simulink subsystem "darm_mechanics"  (R2021a)
settings: Solver=VariableStepAuto  StartTime=0.0  StopTime=10.0  RelTol=1e-3
undefined symbols (not defined in the file): darm, darm_knm, X, Y, Z
libraries: sm_lib x97, darm_library x77
(part 2 of 5)

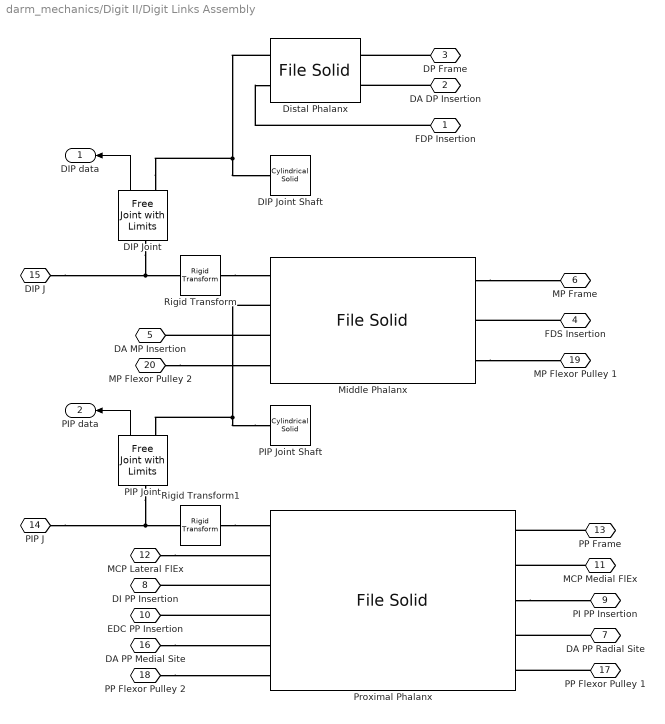
== system darm_mechanics/Digit II/Digit Links Assembly ==
  DIP Joint : darm_library/Free Joint with Limits  joint=digit.dip_joint
  DIP Joint Shaft : sm_lib/Body Elements/Cylindrical Solid  GraphicAmbientColor=[0.15 0.15 0.15 1.0]  BasedOnType=Density  CenterOfMass=[0 0 0]  CenterOfMassUnits=m  GraphicDiffuseColor=[0.5 0.5 0.5]  CylinderLength=digit.dip_joint_shaft_length  CylinderLengthUnits=m  CylinderRadius=digit.dip_joint_shaft_radius  CylinderRadiusUnits=m  Density=darm.link_density  DensityUnits=kg/m^3  DoExposeReferenceFrame=on  GraphicEmissiveColor=[0.0 0.0 0.0 1.0]  ExportEntireGeometry=off  SerializedFrames=<Frames/>  MarkerShape=Sphere  MarkerSize=10  GraphicType=FromGeometry  InertiaType=CalculateFromGeometry  Mass=1  MassUnits=kg  MomentsOfInertia=[1 1 1]  MomentsOfInertiaUnits=kg*m^2  GraphicOpacity=1.0  ProductsOfInertia=[0 0 0]  ProductsOfInertiaUnits=kg*m^2  GraphicShininess=75  GraphicSpecularColor=[0.5 0.5 0.5 1.0]  GraphicVisPropType=SimpleVisualProperties
  Distal Phalanx : sm_lib/Body Elements/File Solid  ExtGeomFileName=C:\Users\Daniel Adejumo\Documents\MATLAB\DARM\Geometry Models and FEA\Models\CAD\Phalanges\Phalanges II\Distal Phalanx II.step  UnitType=FromFile  ExtGeomFileUnits=m  StepReaderType=HEX  ExportConvexHullGeometry=off  InertiaType=CalculateFromGeometry  Mass=1  MassUnits=kg  CenterOfMass=[0 0 0]  CenterOfMassUnits=m  MomentsOfInertia=[1 1 1]  MomentsOfInertiaUnits=kg*m^2  ProductsOfInertia=[0 0 0]  ProductsOfInertiaUnits=kg*m^2  BasedOnType=Density  Density=darm.link_density  DensityUnits=kg/m^3  DoExposeReferenceFrame=on  SerializedFrames=<Frames><Frame><Id>Frame1</Id><Value><Name>J</Name><Origin><Source>ReferenceFrame</Source><FeatureName></FeatureName></Origin><PrimaryAxis><DefinedDirection>+Z</DefinedDirection><Source>ReferenceFrame</Source><SourceDirection>+X</SourceDirection><FeatureName></FeatureName></PrimaryAxis><SecondaryAxis><DefinedDirection>+X</DefinedDirection><Source>ReferenceFrame</Source><SourceDirection>-Z</SourceDirection><FeatureName></FeatureName></SecondaryAxis></Value></Frame><Frame><Id>Frame2</Id><Value><Name>FDP M</Name><Origin><Source>GeometricFeature</Source><FeatureName>circular curve 129</FeatureName></Origin><PrimaryAxis><DefinedDirection>+Z</DefinedDirection><Source>ReferenceFrame</Source><SourceDirection>+Z</SourceDirection><FeatureName></FeatureName></PrimaryAxis><SecondaryAxis><DefinedDirection>+X</DefinedDirection><Source>ReferenceFrame</Source><SourceDirection>+X</SourceDirection><FeatureName></FeatureName></SecondaryAxis></Value></Frame><Frame><Id>Frame3</Id><Value><Name>ED M</Name><Origin><Source>GeometricFeature</Source><FeatureName>circular curve 131</FeatureName></Origin><PrimaryAxis><DefinedDirection>+Z</DefinedDirection><Source>ReferenceFrame</Source><SourceDirection>+Z</SourceDirection><FeatureName></FeatureName></PrimaryAxis><SecondaryAxis><DefinedDirection>+X</DefinedDirection><Source>ReferenceFrame</Source><SourceDirection>+X</SourceDirection><FeatureName></FeatureName></SecondaryAxis></Value></Frame></Frames>  GraphicType=FromGeometry  MarkerShape=Sphere  MarkerSize=10  GraphicVisPropType=SimpleVisualProperties  GraphicDiffuseColor=[0.5 0.5 0.5]  GraphicSpecularColor=[0.5 0.5 0.5 1.0]  GraphicAmbientColor=[0.15 0.15 0.15 1.0]  GraphicEmissiveColor=[0.0 0.0 0.0 1.0]  GraphicShininess=75  GraphicOpacity=1.0
  Middle Phalanx : sm_lib/Body Elements/File Solid  ExtGeomFileName=C:\Users\Daniel Adejumo\Documents\MATLAB\DARM\Geometry Models and FEA\Models\CAD\Phalanges\Phalanges II\Middle Phalanx II.step  UnitType=FromFile  ExtGeomFileUnits=m  StepReaderType=HEX  ExportConvexHullGeometry=off  InertiaType=CalculateFromGeometry  Mass=1  MassUnits=kg  CenterOfMass=[0 0 0]  CenterOfMassUnits=m  MomentsOfInertia=[1 1 1]  MomentsOfInertiaUnits=kg*m^2  ProductsOfInertia=[0 0 0]  ProductsOfInertiaUnits=kg*m^2  BasedOnType=Density  Density=darm.link_density  DensityUnits=kg/m^3  DoExposeReferenceFrame=on  SerializedFrames=<Frames><Frame><Id>Frame2</Id><Value><Name>DIP J*</Name><Origin><Source>GeometricFeature</Source><FeatureName>circular curve 214</FeatureName></Origin><PrimaryAxis><DefinedDirection>+Z</DefinedDirection><Source>ReferenceFrame</Source><SourceDirection>+X</SourceDirection><FeatureName></FeatureName></PrimaryAxis><SecondaryAxis><DefinedDirection>+X</DefinedDirection><Source>ReferenceFrame</Source><SourceDirection>-Z</SourceDirection><FeatureName></FeatureName></SecondaryAxis></Value></Frame><Frame><Id>Frame3</Id><Value><Name>PIP J</Name><Origin><Source>ReferenceFrame</Source><FeatureName></FeatureName></Origin><PrimaryAxis><DefinedDirection>+Z</DefinedDirection><Source>ReferenceFrame</Source><SourceDirection>+X</SourceDirection><FeatureName></FeatureName></PrimaryAxis><SecondaryAxis><DefinedDirection>+X</DefinedDirection><Source>ReferenceFrame</Source><SourceDirection>-Z</SourceDirection><FeatureName></FeatureName></SecondaryAxis></Value></Frame><Frame><Id>Frame4</Id><Value><Name>FDS M</Name><Origin><Source>GeometricFeature</Source><FeatureName>circular curve 209</FeatureName></Origin><PrimaryAxis><DefinedDirection>+Z</DefinedDirection><Source>ReferenceFrame</Source><SourceDirection>+Z</SourceDirection><FeatureName></FeatureName></PrimaryAxis><SecondaryAxis><DefinedDirection>+X</DefinedDirection><Source>ReferenceFrame</Source><SourceDirection>+X</SourceDirection><FeatureName></FeatureName></SecondaryAxis></Value></Frame><Frame><Id>Frame5</Id><Value><Name>ED M</Name><Origin><Source>GeometricFeature</Source><FeatureName>circular curve 205</FeatureName></Origin><PrimaryAxis><DefinedDirection>+Z</DefinedDirection><Source>ReferenceFrame</Source><SourceDirection>+Z</SourceDirection><FeatureName></FeatureName></PrimaryAxis><SecondaryAxis><DefinedDirection>+X</DefinedDirection><Source>ReferenceFrame</Source><SourceDirection>+X</SourceDirection><FeatureName></FeatureName></SecondaryAxis></Value></Frame><Frame><Id>Frame6</Id><Value><Name>Flexor Pulley 1</Name><Origin><Source>GeometricFeature</Source><FeatureName>point 616</FeatureName></Origin><PrimaryAxis><DefinedDirection>+Z</DefinedDirection><Source>ReferenceFrame</Source><SourceDirection>+Z</SourceDirection><FeatureName></FeatureName></PrimaryAxis><SecondaryAxis><DefinedDirection>+X</DefinedDirection><Source>ReferenceFrame</Source><SourceDirection>+X</SourceDirection><FeatureName></FeatureName></SecondaryAxis></Value></Frame><Frame><Id>Frame7</Id><Value><Name>Flexor Pulley 2</Name><Origin><Source>GeometricFeature</Source><FeatureName>segment 75</FeatureName></Origin><PrimaryAxis><DefinedDirection>+Z</DefinedDirection><Source>ReferenceFrame</Source><SourceDirection>+Z</SourceDirection><FeatureName></FeatureName></PrimaryAxis><SecondaryAxis><DefinedDirection>+X</DefinedDirection><Source>ReferenceFrame</Source><SourceDirection>+X</SourceDirection><FeatureName></FeatureName></SecondaryAxis></Value></Frame></Frames>  GraphicType=FromGeometry  MarkerShape=Sphere  MarkerSize=10  GraphicVisPropType=SimpleVisualProperties  GraphicDiffuseColor=[0.5 0.5 0.5]  GraphicSpecularColor=[0.5 0.5 0.5 1.0]  GraphicAmbientColor=[0.15 0.15 0.15 1.0]  GraphicEmissiveColor=[0.0 0.0 0.0 1.0]  GraphicShininess=75  GraphicOpacity=1.0
  PIP Joint : darm_library/Free Joint with Limits  joint=digit.pip_joint
  PIP Joint Shaft : sm_lib/Body Elements/Cylindrical Solid  GraphicAmbientColor=[0.15 0.15 0.15 1.0]  BasedOnType=Density  CenterOfMass=[0 0 0]  CenterOfMassUnits=m  GraphicDiffuseColor=[0.5 0.5 0.5]  CylinderLength=digit.pip_joint_shaft_length  CylinderLengthUnits=m  CylinderRadius=digit.pip_joint_shaft_radius  CylinderRadiusUnits=m  Density=darm.link_density  DensityUnits=kg/m^3  DoExposeReferenceFrame=on  GraphicEmissiveColor=[0.0 0.0 0.0 1.0]  ExportEntireGeometry=off  SerializedFrames=<Frames/>  MarkerShape=Sphere  MarkerSize=10  GraphicType=FromGeometry  InertiaType=CalculateFromGeometry  Mass=1  MassUnits=kg  MomentsOfInertia=[1 1 1]  MomentsOfInertiaUnits=kg*m^2  GraphicOpacity=1.0  ProductsOfInertia=[0 0 0]  ProductsOfInertiaUnits=kg*m^2  GraphicShininess=75  GraphicSpecularColor=[0.5 0.5 0.5 1.0]  GraphicVisPropType=SimpleVisualProperties
  Proximal Phalanx : sm_lib/Body Elements/File Solid  ExtGeomFileName=C:\Users\Daniel Adejumo\Documents\MATLAB\DARM\Geometry Models and FEA\Models\CAD\Phalanges\Phalanges II\Proximal Phalanx II.step  UnitType=FromFile  ExtGeomFileUnits=m  StepReaderType=HEX  ExportConvexHullGeometry=off  InertiaType=CalculateFromGeometry  Mass=1  MassUnits=kg  CenterOfMass=[0 0 0]  CenterOfMassUnits=m  MomentsOfInertia=[1 1 1]  MomentsOfInertiaUnits=kg*m^2  ProductsOfInertia=[0 0 0]  ProductsOfInertiaUnits=kg*m^2  BasedOnType=Density  Density=darm.link_density  DensityUnits=kg/m^3  DoExposeReferenceFrame=on  SerializedFrames=<Frames><Frame><Id>Frame1</Id><Value><Name>PIP J*</Name><Origin><Source>GeometricFeature</Source><FeatureName>circular curve 137</FeatureName></Origin><PrimaryAxis><DefinedDirection>+Z</DefinedDirection><Source>ReferenceFrame</Source><SourceDirection>+X</SourceDirection><FeatureName></FeatureName></PrimaryAxis><SecondaryAxis><DefinedDirection>+X</DefinedDirection><Source>ReferenceFrame</Source><SourceDirection>-Z</SourceDirection><FeatureName></FeatureName></SecondaryAxis></Value></Frame><Frame><Id>Frame2</Id><Value><Name>MCP Lateral FlEx J</Name><Origin><Source>GeometricFeature</Source><FeatureName>circular curve 354</FeatureName></Origin><PrimaryAxis><DefinedDirection>+Z</DefinedDirection><Source>ReferenceFrame</Source><SourceDirection>+X</SourceDirection><FeatureName></FeatureName></PrimaryAxis><SecondaryAxis><DefinedDirection>+X</DefinedDirection><Source>ReferenceFrame</Source><SourceDirection>-Z</SourceDirection><FeatureName></FeatureName></SecondaryAxis></Value></Frame><Frame><Id>Frame3</Id><Value><Name>MCP Medial FlEx J</Name><Origin><Source>GeometricFeature</Source><FeatureName>circular curve 157</FeatureName></Origin><PrimaryAxis><DefinedDirection>+Z</DefinedDirection><Source>ReferenceFrame</Source><SourceDirection>-X</SourceDirection><FeatureName></FeatureName></PrimaryAxis><SecondaryAxis><DefinedDirection>+X</DefinedDirection><Source>ReferenceFrame</Source><SourceDirection>-Z</SourceDirection><FeatureName></FeatureName></SecondaryAxis></Value></Frame><Frame><Id>Frame4</Id><Value><Name>DI M</Name><Origin><Source>GeometricFeature</Source><FeatureName>circular curve 38</FeatureName></Origin><PrimaryAxis><DefinedDirection>+Z</DefinedDirection><Source>ReferenceFrame</Source><SourceDirection>+Z</SourceDirection><FeatureName></FeatureName></PrimaryAxis><SecondaryAxis><DefinedDirection>+X</DefinedDirection><Source>ReferenceFrame</Source><SourceDirection>+X</SourceDirection><FeatureName></FeatureName></SecondaryAxis></Value></Frame><Frame><Id>Frame5</Id><Value><Name>PI M</Name><Origin><Source>GeometricFeature</Source><FeatureName>circular curve 17</FeatureName></Origin><PrimaryAxis><DefinedDirection>+Z</DefinedDirection><Source>ReferenceFrame</Source><SourceDirection>+Z</SourceDirection><FeatureName></FeatureName></PrimaryAxis><SecondaryAxis><DefinedDirection>+X</DefinedDirection><Source>ReferenceFrame</Source><SourceDirection>+X</SourceDirection><FeatureName></FeatureName></SecondaryAxis></Value></Frame><Frame><Id>Frame6</Id><Value><Name>EDC M</Name><Origin><Source>GeometricFeature</Source><FeatureName>circular curve 129</FeatureName></Origin><PrimaryAxis><DefinedDirection>+Z</DefinedDirection><Source>ReferenceFrame</Source><SourceDirection>+Z</SourceDirection><FeatureName></FeatureName></PrimaryAxis><SecondaryAxis><DefinedDirection>+X</DefinedDirection><Source>ReferenceFrame</Source><SourceDirection>+X</SourceDirection><FeatureName></FeatureName></SecondaryAxis></Value></Frame><Frame><Id>Frame7</Id><Value><Name>DA Radial Site</Name><Origin><Source>GeometricFeature</Source><FeatureName>point 850</FeatureName></Origin><PrimaryAxis><DefinedDirection>+Z</DefinedDirection><Source>ReferenceFrame</Source><SourceDirection>+Z</SourceDirection><FeatureName></FeatureName></PrimaryAxis><SecondaryAxis><DefinedDirection>+X</DefinedDirection><Source>ReferenceFrame</Source><SourceDirection>+X</SourceDirection><FeatureName></FeatureName></SecondaryAxis></Value></Frame><Frame><Id>Frame8</Id><Value><Name>DA Medial Site</Name><Origin><Source>GeometricFeature</Source><FeatureName>point 880</FeatureName></Origin><PrimaryAxis><DefinedDirection>+Z</DefinedDirection><Source>ReferenceFrame</Source><SourceDirection>+Z</SourceDirection><FeatureName></FeatureName></PrimaryAxis><SecondaryAxis><DefinedDirection>+X</DefinedDirection><Source>ReferenceFrame</Source><SourceDirection>+X</SourceDirection><FeatureName></FeatureName></SecondaryAxis></Value></Frame><Frame><Id>Frame9</Id><Value><Name>Flexor Pulley 1</Name><Origin><Source>GeometricFeature</Source><FeatureName>segment 120</FeatureName></Origin><PrimaryAxis><DefinedDirection>+Z</DefinedDirection><Source>ReferenceFrame</Source><SourceDirection>+Z</SourceDirection><FeatureName></FeatureName></PrimaryAxis><SecondaryAxis><DefinedDirection>+X</DefinedDirection><Source>ReferenceFrame</Source><SourceDirection>+X</SourceDirection><FeatureName></FeatureName></SecondaryAxis></Value></Frame><Frame><Id>Frame10</Id><Value><Name>Flexor Pulley 2</Name><Origin><Source>GeometricFeature</Source><FeatureName>segment 123</FeatureName></Origin><PrimaryAxis><DefinedDirection>+Z</DefinedDirection><Source>ReferenceFrame</Source><SourceDirection>+Z</SourceDirection><FeatureName></FeatureName></PrimaryAxis><SecondaryAxis><DefinedDirection>+X</DefinedDirection><Source>ReferenceFrame</Source><SourceDirection>+X</SourceDirection><FeatureName></FeatureName></SecondaryAxis></Value></Frame></Frames>  GraphicType=FromGeometry  MarkerShape=Sphere  MarkerSize=10  GraphicVisPropType=SimpleVisualProperties  GraphicDiffuseColor=[0.5 0.5 0.5]  GraphicSpecularColor=[0.5 0.5 0.5 1.0]  GraphicAmbientColor=[0.15 0.15 0.15 1.0]  GraphicEmissiveColor=[0.0 0.0 0.0 1.0]  GraphicShininess=75  GraphicOpacity=1.0
  Rigid Transform : sm_lib/Frames and Transforms/Rigid Transform  TranslationMethod=StandardAxis  TranslationStandardOffset=digit.dip_joint_length/4  TranslationLengthUnit=m  TranslationStandardAxis=+Z  TranslationCartesianOffset=[0 0 0]  TranslationROffset=0  TranslationROffsetUnits=m  TranslationZOffset=0  TranslationZOffsetUnits=m  TranslationThetaOffset=0  TranslationThetaOffsetUnits=deg  RotationMethod=None  RotationAngleUnits=deg  RotationStandardAxis=+Z  RotationAngle=0.0  RotationArbitraryAxis=[0 0 1]  FollAlignAxisA=+X  BaseAlignAxisA=+Y  FollAlignAxisB=+Y  BaseAlignAxisB=+Z  RotationSequenceAxes=FollowerAxes  RotationSequence=XYX  RotationSequenceAngles=[0 0 0]  RotationSequenceAnglesUnits=deg  RotationMatrix=[1 0 0; 0 1 0; 0 0 1]
  Rigid Transform1 : sm_lib/Frames and Transforms/Rigid Transform  TranslationMethod=StandardAxis  TranslationStandardOffset=digit.pip_joint_length/4  TranslationLengthUnit=m  TranslationStandardAxis=+Z  TranslationCartesianOffset=[0 0 0]  TranslationROffset=0  TranslationROffsetUnits=m  TranslationZOffset=0  TranslationZOffsetUnits=m  TranslationThetaOffset=0  TranslationThetaOffsetUnits=deg  RotationMethod=None  RotationAngleUnits=deg  RotationStandardAxis=+Z  RotationAngle=0.0  RotationArbitraryAxis=[0 0 1]  FollAlignAxisA=+X  BaseAlignAxisA=+Y  FollAlignAxisB=+Y  BaseAlignAxisB=+Z  RotationSequenceAxes=FollowerAxes  RotationSequence=XYX  RotationSequenceAngles=[0 0 0]  RotationSequenceAnglesUnits=deg  RotationMatrix=[1 0 0; 0 1 0; 0 0 1]
  FDP Insertion : PMIOPort  Side=Left
  DA DP Insertion : PMIOPort  Port=2  Side=Left
  DP Frame : PMIOPort  Port=3  Side=Right
  FDS Insertion : PMIOPort  Port=4  Side=Left
  DA MP Insertion : PMIOPort  Port=5  Side=Left
  MP Frame : PMIOPort  Port=6  Side=Right
  DA PP Radial Site : PMIOPort  Port=7  Side=Left
  DI PP Insertion : PMIOPort  Port=8  Side=Left
  PI PP Insertion : PMIOPort  Port=9  Side=Left
  EDC PP Insertion : PMIOPort  Port=10  Side=Left
  MCP Medial FlEx : PMIOPort  Port=11  Side=Right
  MCP Lateral FlEx : PMIOPort  Port=12  Side=Right
  PP Frame : PMIOPort  Port=13  Side=Right
  PIP J : PMIOPort  Port=14  Side=Left
  DIP J : PMIOPort  Port=15  Side=Left
  DA PP Medial Site : PMIOPort  Port=16  Side=Left
  PP Flexor Pulley 1 : PMIOPort  Port=17  Side=Left
  PP Flexor Pulley 2 : PMIOPort  Port=18  Side=Left
  MP Flexor Pulley 1 : PMIOPort  Port=19  Side=Left
  MP Flexor Pulley 2 : PMIOPort  Port=20  Side=Left
  DIP data : Outport
  PIP data : Outport  Port=2
  wires:
  PIP Joint/1 -> PIP data/1
  DIP Joint/1 -> DIP data/1
  connections:
  MP Flexor Pulley 2/RConn1 -- Middle Phalanx/LConn4
  Middle Phalanx/RConn3 -- MP Flexor Pulley 1/RConn1
  PP Flexor Pulley 2/RConn1 -- Proximal Phalanx/LConn6
  PP Flexor Pulley 1/RConn1 -- Proximal Phalanx/RConn5
  DA PP Medial Site/RConn1 -- Proximal Phalanx/LConn5
  DIP Joint/RConn1 -- DIP Joint Shaft/RConn1 -- Distal Phalanx/LConn1
  Rigid Transform/LConn1 -- Middle Phalanx/LConn1
  DIP Joint/LConn1 -- Rigid Transform/RConn1 -- DIP J/RConn1
  PP Frame/RConn1 -- Proximal Phalanx/RConn1
  PIP Joint Shaft/RConn1 -- PIP Joint/RConn1 -- Middle Phalanx/LConn2
  Rigid Transform1/LConn1 -- Proximal Phalanx/LConn1
  PIP Joint/LConn1 -- Rigid Transform1/RConn1 -- PIP J/RConn1
  MCP Lateral FlEx/RConn1 -- Proximal Phalanx/LConn2
  MCP Medial FlEx/RConn1 -- Proximal Phalanx/RConn2
  DA DP Insertion/RConn1 -- Distal Phalanx/RConn2
  FDP Insertion/RConn1 -- Distal Phalanx/LConn2
  Middle Phalanx/LConn3 -- DA MP Insertion/RConn1
  FDS Insertion/RConn1 -- Middle Phalanx/RConn2
  DP Frame/RConn1 -- Distal Phalanx/RConn1
  Middle Phalanx/RConn1 -- MP Frame/RConn1
  Proximal Phalanx/RConn3 -- PI PP Insertion/RConn1
  Proximal Phalanx/LConn3 -- DI PP Insertion/RConn1
  Proximal Phalanx/LConn4 -- EDC PP Insertion/RConn1
  DA PP Radial Site/RConn1 -- Proximal Phalanx/RConn4

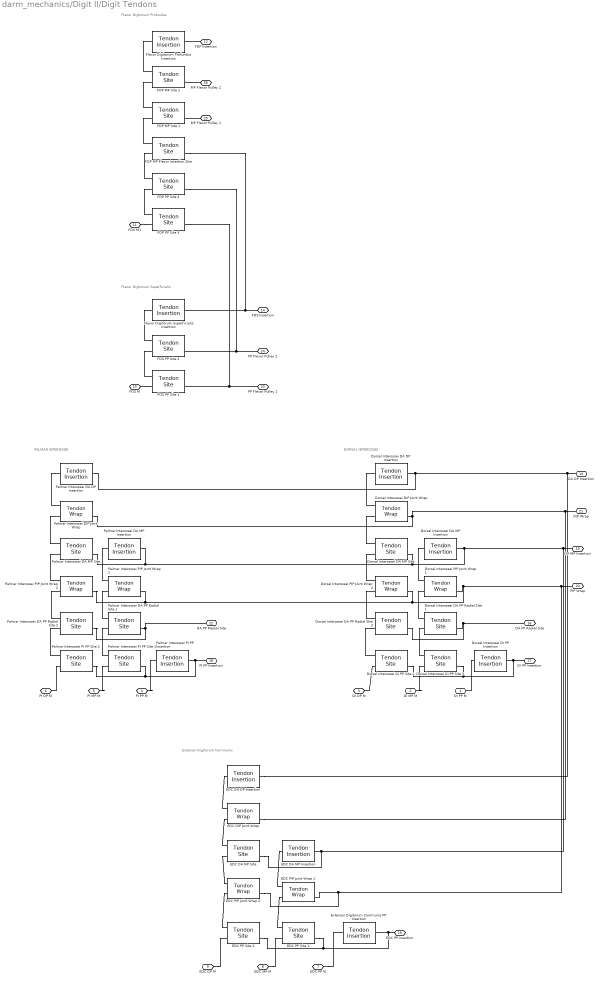
== system darm_mechanics/Digit II/Digit Tendons ==
  note: Flexor Digitorum Profundus
  note: PALMAR INTEROSSEI
  note: DORSAL INTEROSSEI
  note: Extensor Digitorum Communis
  note: Flexor Digitorum Superficialis
  Dorsal Interossei DA DP Insertion : darm_library/Tendon Insertion  muscle=darm.muscles.dorsal_interossei
  Dorsal Interossei DA MP Site : darm_library/Tendon Site  muscle=darm.muscles.dorsal_interossei  site_index=5
  Dorsal Interossei DA PP Radial Site 1 : darm_library/Tendon Site  muscle=darm.muscles.dorsal_interossei  site_index=3
  Dorsal Interossei DA PP Radial Site 2 : darm_library/Tendon Site  muscle=darm.muscles.dorsal_interossei  site_index=3
  Dorsal Interossei DI PP Insertion : darm_library/Tendon Insertion  muscle=darm.muscles.dorsal_interossei
  Dorsal Interossei DI PP Site 1 : darm_library/Tendon Site  muscle=darm.muscles.dorsal_interossei  site_index=1
  Dorsal Interossei DI PP Site 2 : darm_library/Tendon Site  muscle=darm.muscles.dorsal_interossei  site_index=1
  Dorsal Interossei DIP Joint Wrap : darm_library/Tendon Wrap  muscle=darm.muscles.dorsal_interossei  wrap_index=2  flip=off
  Dorsal Interossei PIP Joint Wrap 1 : darm_library/Tendon Wrap  muscle=darm.muscles.dorsal_interossei  wrap_index=1  flip=off
  Dorsal Interossei PIP Joint Wrap 2 : darm_library/Tendon Wrap  muscle=darm.muscles.dorsal_interossei  wrap_index=1  flip=off
  Dorsal Interossei DA MP Insertion : darm_library/Tendon Insertion  muscle=darm.muscles.dorsal_interossei
  EDC DA DP Insertion : darm_library/Tendon Insertion  muscle=darm.muscles.extensor_digitorum
  EDC DA MP Site : darm_library/Tendon Site  muscle=darm.muscles.extensor_digitorum  site_index=7
  EDC DIP Joint Wrap : darm_library/Tendon Wrap  muscle=darm.muscles.extensor_digitorum  wrap_index=4  flip=off
  EDC PIP Joint Wrap 1 : darm_library/Tendon Wrap  muscle=darm.muscles.extensor_digitorum  wrap_index=3  flip=off
  EDC PIP Joint Wrap 2 : darm_library/Tendon Wrap  muscle=darm.muscles.extensor_digitorum  wrap_index=3  flip=off
  EDC PP Site 1 : darm_library/Tendon Site  muscle=darm.muscles.extensor_digitorum  site_index=5
  EDC PP Site 2 : darm_library/Tendon Site  muscle=darm.muscles.extensor_digitorum  site_index=5
  EDC DA MP Insertion : darm_library/Tendon Insertion  muscle=darm.muscles.extensor_digitorum
  Extensor Digitorum Communis PP Insertion : darm_library/Tendon Insertion  muscle=darm.muscles.extensor_digitorum
  FDP MP Flexor Insertion Site : darm_library/Tendon Site  muscle=darm.muscles.flexor_digitorum_profundus  site_index=11
  FDP MP Site 1 : darm_library/Tendon Site  muscle=darm.muscles.flexor_digitorum_profundus  site_index=13
  FDP MP Site 2 : darm_library/Tendon Site  muscle=darm.muscles.flexor_digitorum_profundus  site_index=15
  FDP PP Site 3 : darm_library/Tendon Site  muscle=darm.muscles.flexor_digitorum_profundus  site_index=7
  FDP PP Site 4 : darm_library/Tendon Site  muscle=darm.muscles.flexor_digitorum_profundus  site_index=9
  FDS PP Site 1 : darm_library/Tendon Site  muscle=darm.muscles.flexor_digitorum_superficialis  site_index=7
  FDS PP Site 2 : darm_library/Tendon Site  muscle=darm.muscles.flexor_digitorum_superficialis  site_index=9
  Flexor Digitorum Profundus Insertion : darm_library/Tendon Insertion  muscle=darm.muscles.flexor_digitorum_profundus
  Flexor Digitorum Superficialis Insertion : darm_library/Tendon Insertion  muscle=darm.muscles.flexor_digitorum_superficialis
  Palmar Interossei DA DP Insertion : darm_library/Tendon Insertion  muscle=darm.muscles.palmar_interossei
  Palmar Interossei DA MP Site : darm_library/Tendon Site  muscle=darm.muscles.palmar_interossei  site_index=5
  Palmar Interossei DA PP Radial Site 1 : darm_library/Tendon Site  muscle=darm.muscles.palmar_interossei  site_index=3
  Palmar Interossei DA PP Radial Site 2 : darm_library/Tendon Site  muscle=darm.muscles.palmar_interossei  site_index=3
  Palmar Interossei DIP Joint Wrap : darm_library/Tendon Wrap  muscle=darm.muscles.palmar_interossei  wrap_index=2  flip=off
  Palmar Interossei PI PP Insertion : darm_library/Tendon Insertion  muscle=darm.muscles.palmar_interossei
  Palmar Interossei PI PP Site 1 : darm_library/Tendon Site  muscle=darm.muscles.palmar_interossei  site_index=1
  Palmar Interossei PI PP Site 2 : darm_library/Tendon Site  muscle=darm.muscles.palmar_interossei  site_index=1
  Palmar Interossei PIP Joint Wrap 1 : darm_library/Tendon Wrap  muscle=darm.muscles.palmar_interossei  wrap_index=1  flip=off
  "Palmar Interossei PIP Joint Wrap 2 " : darm_library/Tendon Wrap  muscle=darm.muscles.palmar_interossei  wrap_index=1  flip=off
  Palmar Interossei DA MP Insertion : darm_library/Tendon Insertion  muscle=darm.muscles.palmar_interossei
  DI PP M : PMIOPort  Side=Left
  DI MP M : PMIOPort  Port=2  Side=Left
  DI DP M : PMIOPort  Port=3  Side=Left
  PI PP M : PMIOPort  Port=4  Side=Left
  PI MP M : PMIOPort  Port=5  Side=Left
  PI DP M : PMIOPort  Port=6  Side=Left
  EDC PP M : PMIOPort  Port=7  Side=Left
  EDC MP M : PMIOPort  Port=8  Side=Left
  EDC DP M : PMIOPort  Port=9  Side=Left
  FDS M : PMIOPort  Port=10  Side=Left
  FDS M1 : PMIOPort  Port=11  Side=Left
  FDP Insertion : PMIOPort  Port=12  Side=Right
  DA DP Insertion : PMIOPort  Port=13  Side=Right
  FDS Insertion : PMIOPort  Port=14  Side=Right
  DA MP Insertion : PMIOPort  Port=15  Side=Right
  DA PP Radial Site : PMIOPort  Port=16  Side=Right
  DI PP Insertion : PMIOPort  Port=17  Side=Right
  PI PP Insertion : PMIOPort  Port=18  Side=Right
  EDC PP Insertion : PMIOPort  Port=19  Side=Right
  PIP Wrap : PMIOPort  Port=20  Side=Right
  DIP Wrap : PMIOPort  Port=21  Side=Right
  DA PP Medial Site : PMIOPort  Port=22  Side=Right
  PP Flexor Pulley 1 : PMIOPort  Port=23  Side=Right
  PP Flexor Pulley 2 : PMIOPort  Port=24  Side=Right
  MP Flexor Pulley 1 : PMIOPort  Port=25  Side=Right
  MP Flexor Pulley 2 : PMIOPort  Port=26  Side=Right
  connections:
  MP Flexor Pulley 2/RConn1 -- FDP MP Site 2/RConn1
  MP Flexor Pulley 1/RConn1 -- FDP MP Site 1/RConn1
  FDP MP Site 2/LConn1 -- Flexor Digitorum Profundus Insertion/RConn1
  FDP MP Site 1/LConn1 -- FDP MP Site 2/LConn2
  FDP MP Flexor Insertion Site/LConn1 -- FDP MP Site 1/LConn2
  FDP PP Site 4/LConn1 -- FDP MP Flexor Insertion Site/LConn2
  FDP Insertion/RConn1 -- Flexor Digitorum Profundus Insertion/LConn1
  FDS M1/RConn1 -- FDP PP Site 3/LConn2
  FDP PP Site 3/LConn1 -- FDP PP Site 4/LConn2
  FDP PP Site 3/RConn1 -- PP Flexor Pulley 1/RConn1 -- FDS PP Site 1/RConn1
  FDP PP Site 4/RConn1 -- PP Flexor Pulley 2/RConn1 -- FDS PP Site 2/RConn1
  FDS PP Site 1/LConn1 -- FDS PP Site 2/LConn2
  FDS M/RConn1 -- FDS PP Site 1/LConn2
  FDP MP Flexor Insertion Site/RConn1 -- FDS Insertion/RConn1 -- Flexor Digitorum Superficialis Insertion/LConn1
  FDS PP Site 2/LConn1 -- Flexor Digitorum Superficialis Insertion/RConn1
  EDC DIP Joint Wrap/LConn1 -- EDC DA DP Insertion/RConn1
  EDC DA MP Site/LConn1 -- EDC DIP Joint Wrap/LConn2
  EDC DA MP Site/LConn2 -- EDC PIP Joint Wrap 2/LConn1
  EDC PIP Joint Wrap 1/LConn1 -- EDC DA MP Insertion/RConn1
  EDC PP Site 1/LConn1 -- EDC PIP Joint Wrap 1/LConn2
  EDC PP Site 2/LConn1 -- EDC PIP Joint Wrap 2/LConn2
  EDC PP Site 2/RConn1 -- EDC PP Site 1/RConn1 -- EDC PP Insertion/RConn1 -- Extensor Digitorum Communis PP Insertion/LConn1
  EDC DP M/RConn1 -- EDC PP Site 2/LConn2
  EDC MP M/RConn1 -- EDC PP Site 1/LConn2
  EDC PP M/RConn1 -- Extensor Digitorum Communis PP Insertion/RConn1
  PI PP M/RConn1 -- Palmar Interossei PI PP Insertion/RConn1
  PI MP M/RConn1 -- Palmar Interossei PI PP Site 1/LConn2
  Palmar Interossei PI PP Site 1/LConn1 -- Palmar Interossei DA PP Radial Site 1/LConn2
  PI DP M/RConn1 -- Palmar Interossei PI PP Site 2/LConn2
  Palmar Interossei PI PP Site 2/LConn1 -- Palmar Interossei DA PP Radial Site 2/LConn2
  Palmar Interossei DIP Joint Wrap/LConn2 -- Palmar Interossei DA MP Site/LConn1
  Palmar Interossei DA PP Radial Site 1/LConn1 -- Palmar Interossei PIP Joint Wrap 1/LConn2
  Palmar Interossei DA PP Radial Site 2/LConn1 -- "Palmar Interossei PIP Joint Wrap 2 "/LConn2
  Palmar Interossei PIP Joint Wrap 1/LConn1 -- Palmar Interossei DA MP Insertion/RConn1
  "Palmar Interossei PIP Joint Wrap 2 "/LConn1 -- Palmar Interossei DA MP Site/LConn2
  Palmar Interossei DIP Joint Wrap/LConn1 -- Palmar Interossei DA DP Insertion/RConn1
  Palmar Interossei DA PP Radial Site 1/RConn1 -- Palmar Interossei DA PP Radial Site 2/RConn1 -- DA PP Medial Site/RConn1
  Palmar Interossei PI PP Site 1/RConn1 -- Palmar Interossei PI PP Site 2/RConn1 -- PI PP Insertion/RConn1 -- Palmar Interossei PI PP Insertion/LConn1
  Dorsal Interossei DIP Joint Wrap/RConn1 -- Palmar Interossei DIP Joint Wrap/RConn1 -- EDC DIP Joint Wrap/RConn1 -- DIP Wrap/RConn1
  Dorsal Interossei DIP Joint Wrap/LConn1 -- Dorsal Interossei DA DP Insertion/RConn1
  Dorsal Interossei PIP Joint Wrap 2/LConn1 -- Dorsal Interossei DA MP Site/LConn2
  Dorsal Interossei PIP Joint Wrap 1/LConn1 -- Dorsal Interossei DA MP Insertion/RConn1
  PIP Wrap/RConn1 -- EDC PIP Joint Wrap 1/RConn1 -- EDC PIP Joint Wrap 2/RConn1 -- "Palmar Interossei PIP Joint Wrap 2 "/RConn1 -- Palmar Interossei PIP Joint Wrap 1/RConn1 -- Dorsal Interossei PIP Joint Wrap 2/RConn1 -- Dorsal Interossei PIP Joint Wrap 1/RConn1
  Dorsal Interossei DA PP Radial Site 2/LConn1 -- Dorsal Interossei PIP Joint Wrap 2/LConn2
  Dorsal Interossei DA PP Radial Site 1/LConn1 -- Dorsal Interossei PIP Joint Wrap 1/LConn2
  Dorsal Interossei DA PP Radial Site 1/RConn1 -- DA PP Radial Site/RConn1 -- Dorsal Interossei DA PP Radial Site 2/RConn1
  Dorsal Interossei DIP Joint Wrap/LConn2 -- Dorsal Interossei DA MP Site/LConn1
  Dorsal Interossei DI PP Site 2/LConn1 -- Dorsal Interossei DA PP Radial Site 2/LConn2
  DI DP M/RConn1 -- Dorsal Interossei DI PP Site 2/LConn2
  Dorsal Interossei DI PP Site 1/LConn1 -- Dorsal Interossei DA PP Radial Site 1/LConn2
  DI MP M/RConn1 -- Dorsal Interossei DI PP Site 1/LConn2
  Palmar Interossei DA DP Insertion/LConn1 -- Dorsal Interossei DA DP Insertion/LConn1 -- EDC DA DP Insertion/LConn1 -- DA DP Insertion/RConn1
  Dorsal Interossei DA MP Insertion/LConn1 -- Palmar Interossei DA MP Site/RConn1 -- Palmar Interossei DA MP Insertion/LConn1 -- Dorsal Interossei DA MP Site/RConn1 -- EDC DA MP Insertion/LConn1 -- EDC DA MP Site/RConn1 -- DA MP Insertion/RConn1
  DI PP M/RConn1 -- Dorsal Interossei DI PP Insertion/RConn1
  Dorsal Interossei DI PP Site 2/RConn1 -- Dorsal Interossei DI PP Insertion/LConn1 -- DI PP Insertion/RConn1 -- Dorsal Interossei DI PP Site 1/RConn1

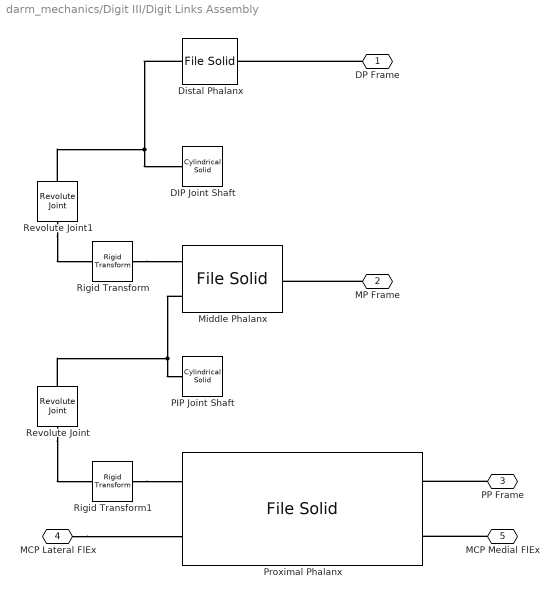
== system darm_mechanics/Digit III/Digit Links Assembly ==
  DIP Joint Shaft : sm_lib/Body Elements/Cylindrical Solid  GraphicAmbientColor=[0.15 0.15 0.15 1.0]  BasedOnType=Density  CenterOfMass=[0 0 0]  CenterOfMassUnits=m  GraphicDiffuseColor=[0.5 0.5 0.5]  CylinderLength=digit.dip_joint_shaft_length  CylinderLengthUnits=m  CylinderRadius=digit.dip_joint_shaft_radius  CylinderRadiusUnits=m  Density=darm_dnm.link_density  DensityUnits=kg/m^3  DoExposeReferenceFrame=on  GraphicEmissiveColor=[0.0 0.0 0.0 1.0]  ExportEntireGeometry=off  SerializedFrames=<Frames/>  MarkerShape=Sphere  MarkerSize=10  GraphicType=FromGeometry  InertiaType=CalculateFromGeometry  Mass=1  MassUnits=kg  MomentsOfInertia=[1 1 1]  MomentsOfInertiaUnits=kg*m^2  GraphicOpacity=1.0  ProductsOfInertia=[0 0 0]  ProductsOfInertiaUnits=kg*m^2  GraphicShininess=75  GraphicSpecularColor=[0.5 0.5 0.5 1.0]  GraphicVisPropType=SimpleVisualProperties
  Distal Phalanx : sm_lib/Body Elements/File Solid  ExtGeomFileName=C:\Users\Daniel Adejumo\Documents\MATLAB\DARM\Geometry Models and FEA\Models\CAD\Phalanges\Phalanges III\Distal Phalanx III.step  UnitType=FromFile  ExtGeomFileUnits=m  StepReaderType=HEX  ExportConvexHullGeometry=off  InertiaType=CalculateFromGeometry  Mass=1  MassUnits=kg  CenterOfMass=[0 0 0]  CenterOfMassUnits=m  MomentsOfInertia=[1 1 1]  MomentsOfInertiaUnits=kg*m^2  ProductsOfInertia=[0 0 0]  ProductsOfInertiaUnits=kg*m^2  BasedOnType=Density  Density=darm_dnm.link_density  DensityUnits=kg/m^3  DoExposeReferenceFrame=on  SerializedFrames=<Frames><Frame><Id>Frame1</Id><Value><Name>J</Name><Origin><Source>ReferenceFrame</Source><FeatureName></FeatureName></Origin><PrimaryAxis><DefinedDirection>+Z</DefinedDirection><Source>ReferenceFrame</Source><SourceDirection>+X</SourceDirection><FeatureName></FeatureName></PrimaryAxis><SecondaryAxis><DefinedDirection>+X</DefinedDirection><Source>ReferenceFrame</Source><SourceDirection>-Z</SourceDirection><FeatureName></FeatureName></SecondaryAxis></Value></Frame></Frames>  GraphicType=FromGeometry  MarkerShape=Sphere  MarkerSize=10  GraphicVisPropType=SimpleVisualProperties  GraphicDiffuseColor=[0.5 0.5 0.5]  GraphicSpecularColor=[0.5 0.5 0.5 1.0]  GraphicAmbientColor=[0.15 0.15 0.15 1.0]  GraphicEmissiveColor=[0.0 0.0 0.0 1.0]  GraphicShininess=75  GraphicOpacity=1.0
  Middle Phalanx : sm_lib/Body Elements/File Solid  ExtGeomFileName=C:\Users\Daniel Adejumo\Documents\MATLAB\DARM\Geometry Models and FEA\Models\CAD\Phalanges\Phalanges III\Middle Phalanx III.step  UnitType=FromFile  ExtGeomFileUnits=m  StepReaderType=HEX  ExportConvexHullGeometry=off  InertiaType=CalculateFromGeometry  Mass=1  MassUnits=kg  CenterOfMass=[0 0 0]  CenterOfMassUnits=m  MomentsOfInertia=[1 1 1]  MomentsOfInertiaUnits=kg*m^2  ProductsOfInertia=[0 0 0]  ProductsOfInertiaUnits=kg*m^2  BasedOnType=Density  Density=darm_dnm.link_density  DensityUnits=kg/m^3  DoExposeReferenceFrame=on  SerializedFrames=<Frames><Frame><Id>Frame2</Id><Value><Name>DIP J*</Name><Origin><Source>GeometricFeature</Source><FeatureName>circular curve 222</FeatureName></Origin><PrimaryAxis><DefinedDirection>+Z</DefinedDirection><Source>ReferenceFrame</Source><SourceDirection>+X</SourceDirection><FeatureName></FeatureName></PrimaryAxis><SecondaryAxis><DefinedDirection>+X</DefinedDirection><Source>ReferenceFrame</Source><SourceDirection>-Z</SourceDirection><FeatureName></FeatureName></SecondaryAxis></Value></Frame><Frame><Id>Frame3</Id><Value><Name>PIP J</Name><Origin><Source>ReferenceFrame</Source><FeatureName></FeatureName></Origin><PrimaryAxis><DefinedDirection>+Z</DefinedDirection><Source>ReferenceFrame</Source><SourceDirection>+X</SourceDirection><FeatureName></FeatureName></PrimaryAxis><SecondaryAxis><DefinedDirection>+X</DefinedDirection><Source>ReferenceFrame</Source><SourceDirection>-Z</SourceDirection><FeatureName></FeatureName></SecondaryAxis></Value></Frame></Frames>  GraphicType=FromGeometry  MarkerShape=Sphere  MarkerSize=10  GraphicVisPropType=SimpleVisualProperties  GraphicDiffuseColor=[0.5 0.5 0.5]  GraphicSpecularColor=[0.5 0.5 0.5 1.0]  GraphicAmbientColor=[0.15 0.15 0.15 1.0]  GraphicEmissiveColor=[0.0 0.0 0.0 1.0]  GraphicShininess=75  GraphicOpacity=1.0
  PIP Joint Shaft : sm_lib/Body Elements/Cylindrical Solid  GraphicAmbientColor=[0.15 0.15 0.15 1.0]  BasedOnType=Density  CenterOfMass=[0 0 0]  CenterOfMassUnits=m  GraphicDiffuseColor=[0.5 0.5 0.5]  CylinderLength=digit.pip_joint_shaft_length  CylinderLengthUnits=m  CylinderRadius=digit.pip_joint_shaft_radius  CylinderRadiusUnits=m  Density=darm_dnm.link_density  DensityUnits=kg/m^3  DoExposeReferenceFrame=on  GraphicEmissiveColor=[0.0 0.0 0.0 1.0]  ExportEntireGeometry=off  SerializedFrames=<Frames/>  MarkerShape=Sphere  MarkerSize=10  GraphicType=FromGeometry  InertiaType=CalculateFromGeometry  Mass=1  MassUnits=kg  MomentsOfInertia=[1 1 1]  MomentsOfInertiaUnits=kg*m^2  GraphicOpacity=1.0  ProductsOfInertia=[0 0 0]  ProductsOfInertiaUnits=kg*m^2  GraphicShininess=75  GraphicSpecularColor=[0.5 0.5 0.5 1.0]  GraphicVisPropType=SimpleVisualProperties
  Proximal Phalanx : sm_lib/Body Elements/File Solid  ExtGeomFileName=C:\Users\Daniel Adejumo\Documents\MATLAB\DARM\Geometry Models and FEA\Models\CAD\Phalanges\Phalanges III\Proximal Phalanx III.step  UnitType=FromFile  ExtGeomFileUnits=m  StepReaderType=HEX  ExportConvexHullGeometry=off  InertiaType=CalculateFromGeometry  Mass=1  MassUnits=kg  CenterOfMass=[0 0 0]  CenterOfMassUnits=m  MomentsOfInertia=[1 1 1]  MomentsOfInertiaUnits=kg*m^2  ProductsOfInertia=[0 0 0]  ProductsOfInertiaUnits=kg*m^2  BasedOnType=Density  Density=darm_dnm.link_density  DensityUnits=kg/m^3  DoExposeReferenceFrame=on  SerializedFrames=<Frames><Frame><Id>Frame1</Id><Value><Name>PIP J*</Name><Origin><Source>GeometricFeature</Source><FeatureName>circular curve 340</FeatureName></Origin><PrimaryAxis><DefinedDirection>+Z</DefinedDirection><Source>ReferenceFrame</Source><SourceDirection>+X</SourceDirection><FeatureName></FeatureName></PrimaryAxis><SecondaryAxis><DefinedDirection>+X</DefinedDirection><Source>ReferenceFrame</Source><SourceDirection>-Z</SourceDirection><FeatureName></FeatureName></SecondaryAxis></Value></Frame><Frame><Id>Frame2</Id><Value><Name>MCP Lateral FlEx J</Name><Origin><Source>GeometricFeature</Source><FeatureName>circular curve 160</FeatureName></Origin><PrimaryAxis><DefinedDirection>+Z</DefinedDirection><Source>ReferenceFrame</Source><SourceDirection>+X</SourceDirection><FeatureName></FeatureName></PrimaryAxis><SecondaryAxis><DefinedDirection>+X</DefinedDirection><Source>ReferenceFrame</Source><SourceDirection>-Z</SourceDirection><FeatureName></FeatureName></SecondaryAxis></Value></Frame><Frame><Id>Frame3</Id><Value><Name>MCP Medial FlEx J</Name><Origin><Source>GeometricFeature</Source><FeatureName>circular curve 333</FeatureName></Origin><PrimaryAxis><DefinedDirection>+Z</DefinedDirection><Source>ReferenceFrame</Source><SourceDirection>-X</SourceDirection><FeatureName></FeatureName></PrimaryAxis><SecondaryAxis><DefinedDirection>+X</DefinedDirection><Source>ReferenceFrame</Source><SourceDirection>-Z</SourceDirection><FeatureName></FeatureName></SecondaryAxis></Value></Frame></Frames>  GraphicType=FromGeometry  MarkerShape=Sphere  MarkerSize=10  GraphicVisPropType=SimpleVisualProperties  GraphicDiffuseColor=[0.5 0.5 0.5]  GraphicSpecularColor=[0.5 0.5 0.5 1.0]  GraphicAmbientColor=[0.15 0.15 0.15 1.0]  GraphicEmissiveColor=[0.0 0.0 0.0 1.0]  GraphicShininess=75  GraphicOpacity=1.0
  Revolute Joint : sm_lib/Joints/Revolute Joint  JointMode=Normal  SenseConstraintForce=off  SenseConstraintForceX=off  SenseConstraintForceY=off  SenseConstraintForceZ=off  SenseConstraintTorque=off  SenseConstraintTorqueX=off  SenseConstraintTorqueY=off  SenseConstraintTorqueZ=off  SenseTotalForce=off  SenseTotalForceX=off  SenseTotalForceY=off  SenseTotalForceZ=off  SenseTotalTorque=off  SenseTotalTorqueX=off  SenseTotalTorqueY=off  SenseTotalTorqueZ=off  CompositeWrenchDir=FollowerOnBase  CompositeWrenchFrame=BaseFrame  EquilibriumPosition=0  EquilibriumPositionUnits=deg  SpringStiffness=0  SpringStiffnessUnits=N*m/deg  DampingCoefficient=0  DampingCoefficientUnits=N*m/(deg/s)  TorqueActuationMode=NoTorque  MotionActuationMode=ComputedMotion  SensePosition=off  SenseVelocity=off  SenseAcceleration=off  SenseTorqueForce=off  SenseLowerLimitTorqueForce=off  SenseUpperLimitTorqueForce=off  LowerLimitSpecify=off  LowerLimitBound=-90  LowerLimitBoundUnits=deg  LowerLimitStiffness=1e4  LowerLimitStiffnessUnits=N*m/deg  LowerLimitDamping=10  LowerLimitDampingUnits=N*m/(deg/s)  LowerLimitTransitionRegionWidth=0.1  LowerLimitTransitionRegionWidthUnits=deg  UpperLimitSpecify=off  UpperLimitBound=90  UpperLimitBoundUnits=deg  UpperLimitStiffness=1e4  UpperLimitStiffnessUnits=N*m/deg  UpperLimitDamping=10  UpperLimitDampingUnits=N*m/(deg/s)  UpperLimitTransitionRegionWidth=0.1  UpperLimitTransitionRegionWidthUnits=deg  PositionTargetSpecify=off  PositionTargetPriority=High  PositionTargetValue=0  PositionTargetValueUnits=deg  VelocityTargetSpecify=off  VelocityTargetPriority=High  VelocityTargetValue=0  VelocityTargetValueUnits=deg/s
  Revolute Joint1 : sm_lib/Joints/Revolute Joint  JointMode=Normal  SenseConstraintForce=off  SenseConstraintForceX=off  SenseConstraintForceY=off  SenseConstraintForceZ=off  SenseConstraintTorque=off  SenseConstraintTorqueX=off  SenseConstraintTorqueY=off  SenseConstraintTorqueZ=off  SenseTotalForce=off  SenseTotalForceX=off  SenseTotalForceY=off  SenseTotalForceZ=off  SenseTotalTorque=off  SenseTotalTorqueX=off  SenseTotalTorqueY=off  SenseTotalTorqueZ=off  CompositeWrenchDir=FollowerOnBase  CompositeWrenchFrame=BaseFrame  EquilibriumPosition=0  EquilibriumPositionUnits=deg  SpringStiffness=0  SpringStiffnessUnits=N*m/deg  DampingCoefficient=0  DampingCoefficientUnits=N*m/(deg/s)  TorqueActuationMode=NoTorque  MotionActuationMode=ComputedMotion  SensePosition=off  SenseVelocity=off  SenseAcceleration=off  SenseTorqueForce=off  SenseLowerLimitTorqueForce=off  SenseUpperLimitTorqueForce=off  LowerLimitSpecify=off  LowerLimitBound=-90  LowerLimitBoundUnits=deg  LowerLimitStiffness=1e4  LowerLimitStiffnessUnits=N*m/deg  LowerLimitDamping=10  LowerLimitDampingUnits=N*m/(deg/s)  LowerLimitTransitionRegionWidth=0.1  LowerLimitTransitionRegionWidthUnits=deg  UpperLimitSpecify=off  UpperLimitBound=90  UpperLimitBoundUnits=deg  UpperLimitStiffness=1e4  UpperLimitStiffnessUnits=N*m/deg  UpperLimitDamping=10  UpperLimitDampingUnits=N*m/(deg/s)  UpperLimitTransitionRegionWidth=0.1  UpperLimitTransitionRegionWidthUnits=deg  PositionTargetSpecify=off  PositionTargetPriority=High  PositionTargetValue=0  PositionTargetValueUnits=deg  VelocityTargetSpecify=off  VelocityTargetPriority=High  VelocityTargetValue=0  VelocityTargetValueUnits=deg/s
  Rigid Transform : sm_lib/Frames and Transforms/Rigid Transform  TranslationMethod=StandardAxis  TranslationStandardOffset=digit.dip_joint_length/4  TranslationLengthUnit=m  TranslationStandardAxis=+Z  TranslationCartesianOffset=[0 0 0]  TranslationROffset=0  TranslationROffsetUnits=m  TranslationZOffset=0  TranslationZOffsetUnits=m  TranslationThetaOffset=0  TranslationThetaOffsetUnits=deg  RotationMethod=None  RotationAngleUnits=deg  RotationStandardAxis=+Z  RotationAngle=0.0  RotationArbitraryAxis=[0 0 1]  FollAlignAxisA=+X  BaseAlignAxisA=+Y  FollAlignAxisB=+Y  BaseAlignAxisB=+Z  RotationSequenceAxes=FollowerAxes  RotationSequence=XYX  RotationSequenceAngles=[0 0 0]  RotationSequenceAnglesUnits=deg  RotationMatrix=[1 0 0; 0 1 0; 0 0 1]
  Rigid Transform1 : sm_lib/Frames and Transforms/Rigid Transform  TranslationMethod=StandardAxis  TranslationStandardOffset=digit.pip_joint_length/4  TranslationLengthUnit=m  TranslationStandardAxis=+Z  TranslationCartesianOffset=[0 0 0]  TranslationROffset=0  TranslationROffsetUnits=m  TranslationZOffset=0  TranslationZOffsetUnits=m  TranslationThetaOffset=0  TranslationThetaOffsetUnits=deg  RotationMethod=None  RotationAngleUnits=deg  RotationStandardAxis=+Z  RotationAngle=0.0  RotationArbitraryAxis=[0 0 1]  FollAlignAxisA=+X  BaseAlignAxisA=+Y  FollAlignAxisB=+Y  BaseAlignAxisB=+Z  RotationSequenceAxes=FollowerAxes  RotationSequence=XYX  RotationSequenceAngles=[0 0 0]  RotationSequenceAnglesUnits=deg  RotationMatrix=[1 0 0; 0 1 0; 0 0 1]
  DP Frame : PMIOPort  Side=Left
  MP Frame : PMIOPort  Port=2  Side=Left
  PP Frame : PMIOPort  Port=3  Side=Left
  MCP Lateral FlEx : PMIOPort  Port=4  Side=Left
  MCP Medial FlEx : PMIOPort  Port=5  Side=Left
  connections:
  MCP Medial FlEx/RConn1 -- Proximal Phalanx/RConn2
  MCP Lateral FlEx/RConn1 -- Proximal Phalanx/LConn2
  Revolute Joint/LConn1 -- Rigid Transform1/RConn1
  Rigid Transform1/LConn1 -- Proximal Phalanx/LConn1
  Revolute Joint/RConn1 -- Middle Phalanx/LConn2 -- PIP Joint Shaft/RConn1
  PP Frame/RConn1 -- Proximal Phalanx/RConn1
  MP Frame/RConn1 -- Middle Phalanx/RConn1
  DP Frame/RConn1 -- Distal Phalanx/RConn1
  Revolute Joint1/LConn1 -- Rigid Transform/RConn1
  Rigid Transform/LConn1 -- Middle Phalanx/LConn1
  Revolute Joint1/RConn1 -- Distal Phalanx/LConn1 -- DIP Joint Shaft/RConn1
